simulink model "SimuPilot"  (R2024b)
settings: Solver=VariableStepAuto  StartTime=0.0  StopTime=10.0  RelTol=1e-3
undefined symbols (not defined in the file or in its folder): aspd_min, gravity, H_INIT, K_D, K_H, K_T, K_V, mass, PTCH2SRV_D, PTCH2SRV_RLL, PTCH2SRV_RMAX_DN, PTCH2SRV_RMAX_UP, PTCH2SRV_TCONST, PTCH_K_I, PTCH_K_P, RLL2SRV_D, RLL2SRV_MAX, RLL2SRV_TCONST, RLL_K_I, RLL_K_P, V_INIT, YAW2SRV_DAMP, YAW2SRV_INT, YAW2SRV_RLL, YAW2SRV_SLIP
settings Model: Creator=sh2323  LastModifiedBy=sh2323

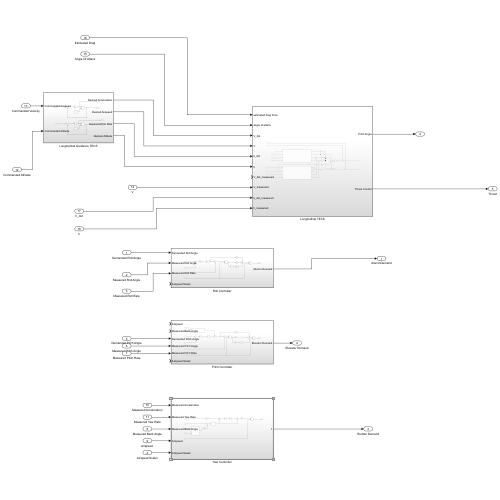
[thumbnail: Simulink's stored preview of the top-level diagram]
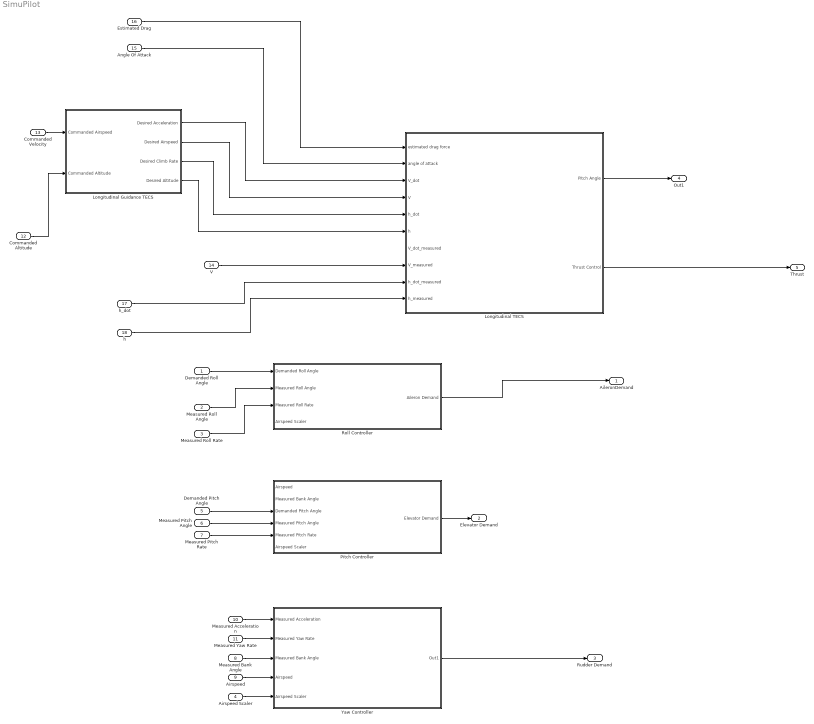
== system SimuPilot ==
  Demanded Roll Angle : Inport
  Measured Roll Angle : Inport  Port=2
  Measured Roll Rate : Inport  Port=3
  Airspeed Scaler : Inport  Port=4
  Demanded Pitch Angle : Inport  Port=5
  Measured Pitch Angle : Inport  Port=6
  Measured Pitch Rate : Inport  Port=7
  Measured Bank Angle : Inport  Port=8
  "Airspeed " : Inport  Port=9
  Measured Acceleration : Inport  Port=10
  Measured Yaw Rate : Inport  Port=11
  Commanded Altitude : Inport  Port=12
  Commanded Velocity : Inport  Port=13
  V : Inport  Port=14
  Angle Of Attack : Inport  Port=15
  Estimated Drag : Inport  Port=16
  h_dot : Inport  Port=17
  h : Inport  Port=18
  Longitudinal Guidance TECS : Subsystem
  Longitudinal TECS : Subsystem
  Pitch Controller : Subsystem
  Roll Controller : Subsystem
  Yaw Controller : Subsystem
  AileronDemand : Outport
  Elevator Demand : Outport  Port=2
  Rudder Demand : Outport  Port=3
  Out1 : Outport  Port=4
  Thrust : Outport  Port=5
  wires:
  Demanded Roll Angle/1 -> Roll Controller/1(Demanded Roll Angle)
  Measured Roll Angle/1 -> Roll Controller/2(Measured Roll Angle)
  Measured Roll Rate/1 -> Roll Controller/3(Measured Roll Rate)
  Roll Controller/1(Aileron Demand) -> AileronDemand/1
  Demanded Pitch Angle/1 -> Pitch Controller/3(Demanded Pitch Angle)
  Measured Pitch Angle/1 -> Pitch Controller/4(Measured Pitch Angle)
  Measured Pitch Rate/1 -> Pitch Controller/5(Measured Pitch Rate)
  Pitch Controller/1(Elevator Demand) -> Elevator Demand/1
  Measured Acceleration/1 -> Yaw Controller/1(Measured Acceleration)
  Measured Yaw Rate/1 -> Yaw Controller/2(Measured Yaw Rate)
  Measured Bank Angle/1 -> Yaw Controller/3(Measured Bank Angle)
  "Airspeed "/1 -> Yaw Controller/4(Airspeed)
  Airspeed Scaler/1 -> Yaw Controller/5(Airspeed Scaler)
  Yaw Controller/1(Out1) -> Rudder Demand/1
  Commanded Velocity/1 -> Longitudinal Guidance TECS/1(Commanded Airspeed)
  Commanded Altitude/1 -> Longitudinal Guidance TECS/2(Commanded Altitude)
  Estimated Drag/1 -> Longitudinal TECS/1(estimated drag force)
  Angle Of Attack/1 -> Longitudinal TECS/2(angle of attack)
  Longitudinal Guidance TECS/1(Desired Acceleration) -> Longitudinal TECS/3(V_dot)
  Longitudinal Guidance TECS/2(Desired Airspeed) -> Longitudinal TECS/4(V)
  Longitudinal Guidance TECS/3(Desired Climb Rate) -> Longitudinal TECS/5(h_dot)
  Longitudinal Guidance TECS/4(Desired Altitude) -> Longitudinal TECS/6(h)
  V/1 -> Longitudinal TECS/8(V_measured)
  h_dot/1 -> Longitudinal TECS/9(h_dot_measured)
  h/1 -> Longitudinal TECS/10(h_measured)
  Longitudinal TECS/1(Pitch Angle) -> Out1/1
  Longitudinal TECS/2(Thrust Control) -> Thrust/1

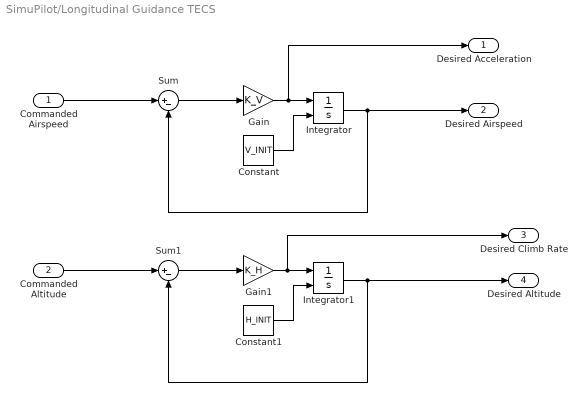
== system SimuPilot/Longitudinal Guidance TECS ==
  Commanded Airspeed : Inport
  Commanded Altitude : Inport  Port=2
  Constant : Constant  Value=V_INIT
  Constant1 : Constant  Value=H_INIT
  Gain : Gain  Gain=K_V
  Gain1 : Gain  Gain=K_H
  Integrator : Integrator  InitialConditionSource=external
  Integrator1 : Integrator  InitialConditionSource=external
  Sum : Sum  Inputs=|+-
  Sum1 : Sum  Inputs=|+-
  Desired Acceleration : Outport
  Desired Airspeed : Outport  Port=2
  Desired Climb Rate : Outport  Port=3
  Desired Altitude : Outport  Port=4
  wires:
  Sum/1 -> Gain/1
  Gain/1 -> Desired Acceleration/1, Integrator/1
  Commanded Altitude/1 -> Sum1/1
  Constant/1 -> Integrator/2
  Integrator1/1 -> Desired Altitude/1, Sum1/2
  Gain1/1 -> Desired Climb Rate/1, Integrator1/1
  Commanded Airspeed/1 -> Sum/1
  Integrator/1 -> Desired Airspeed/1, Sum/2
  Constant1/1 -> Integrator1/2
  Sum1/1 -> Gain1/1

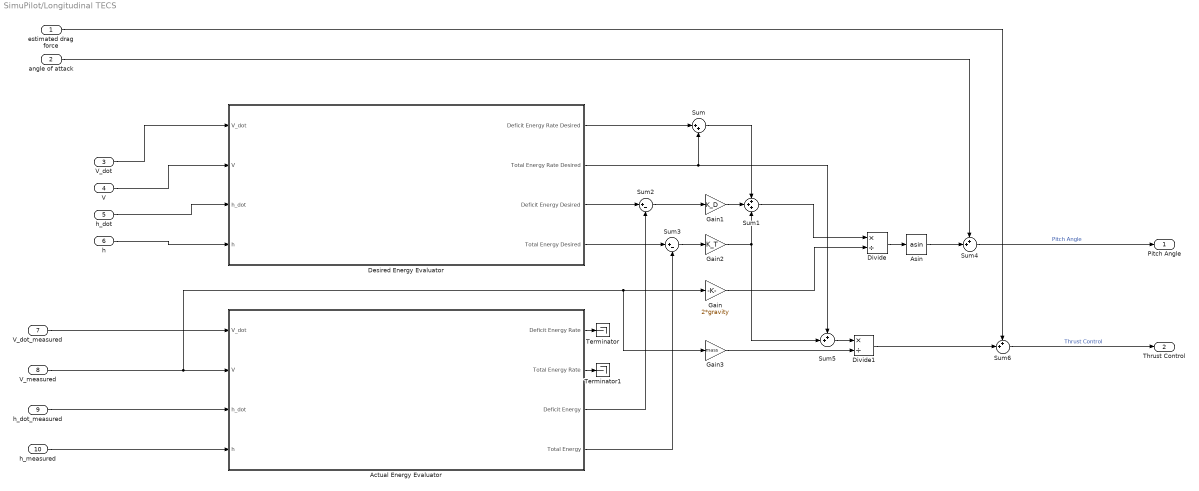
== system SimuPilot/Longitudinal TECS ==
  estimated drag force : Inport
  angle of attack : Inport  Port=2
  V_dot : Inport  Port=3
  V : Inport  Port=4
  h_dot : Inport  Port=5
  h : Inport  Port=6
  V_dot_measured : Inport  Port=7
  V_measured : Inport  Port=8
  h_dot_measured : Inport  Port=9
  h_measured : Inport  Port=10
  Actual Energy Evaluator : Subsystem
  Asin : Trigonometry  Operator=asin
  Desired Energy Evaluator : Subsystem
  Divide : Product  Inputs=*/
  Divide1 : Product  Inputs=*/
  Gain : Gain  Gain=2*gravity
  Gain1 : Gain  Gain=K_D
  Gain2 : Gain  Gain=K_T
  Gain3 : Gain  Gain=mass
  Sum : Sum  Inputs=|++
  Sum1 : Sum  Inputs=+++
  Sum2 : Sum  Inputs=|+-
  Sum3 : Sum  Inputs=|+-
  Sum4 : Sum  Inputs=++|
  Sum5 : Sum  Inputs=++|
  Sum6 : Sum  Inputs=++|
  Terminator : Terminator
  Terminator1 : Terminator
  Pitch Angle : Outport
  Thrust Control : Outport  Port=2
  wires:
  Desired Energy Evaluator/2(Total Energy Rate Desired) -> Sum5/1, Sum/2
  Divide/1 -> Asin/1
  Gain2/1 -> Sum5/2, Sum1/3
  angle of attack/1 -> Sum4/1
  Actual Energy Evaluator/3(Deficit Energy) -> Sum2/2
  V/1 -> Desired Energy Evaluator/2(V)
  Desired Energy Evaluator/3(Deficit Energy Desired) -> Sum2/1
  Sum3/1 -> Gain2/1
  V_measured/1 -> Gain3/1, Gain/1, Actual Energy Evaluator/2(V)
  Actual Energy Evaluator/4(Total Energy) -> Sum3/2
  h_dot_measured/1 -> Actual Energy Evaluator/3(h_dot)
  Sum/1 -> Sum1/1
  Gain/1 -> Divide/2
  Desired Energy Evaluator/1(Deficit Energy Rate Desired) -> Sum/1
  Gain3/1 -> Divide1/2
  Actual Energy Evaluator/1(Deficit Energy Rate) -> Terminator/1
  Divide1/1 -> Sum6/2
  Actual Energy Evaluator/2(Total Energy Rate) -> Terminator1/1
  h/1 -> Desired Energy Evaluator/4(h)
  Desired Energy Evaluator/4(Total Energy Desired) -> Sum3/1
  Sum5/1 -> Divide1/1
  Sum2/1 -> Gain1/1
  Asin/1 -> Sum4/2
  Gain1/1 -> Sum1/2
  Sum1/1 -> Divide/1
  V_dot_measured/1 -> Actual Energy Evaluator/1(V_dot)
  h_dot/1 -> Desired Energy Evaluator/3(h_dot)
  estimated drag force/1 -> Sum6/1
  V_dot/1 -> Desired Energy Evaluator/1(V_dot)
  Sum6/1 -> Thrust Control/1  "Thrust Control"
  h_measured/1 -> Actual Energy Evaluator/4(h)
  Sum4/1 -> Pitch Angle/1  "Pitch Angle"

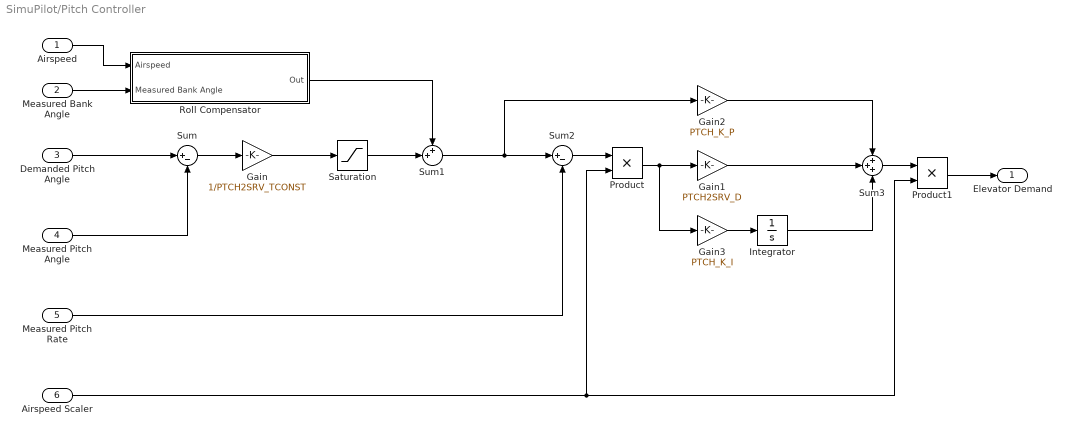
== system SimuPilot/Pitch Controller ==
  Airspeed : Inport
  Measured Bank Angle : Inport  Port=2
  Demanded Pitch Angle : Inport  Port=3
  Measured Pitch Angle : Inport  Port=4
  Measured Pitch Rate : Inport  Port=5
  Airspeed Scaler : Inport  Port=6
  Gain : Gain  Gain=1/PTCH2SRV_TCONST
  Gain1 : Gain  Gain=PTCH2SRV_D
  Gain2 : Gain  Gain=PTCH_K_P
  Gain3 : Gain  Gain=PTCH_K_I
  Integrator : Integrator
  Product : Product
  Product1 : Product
  Roll Compensator : Subsystem
  Saturation : Saturate  UpperLimit=PTCH2SRV_RMAX_UP  LowerLimit=PTCH2SRV_RMAX_DN
  Sum : Sum  Inputs=|+-
  Sum1 : Sum  Inputs=++|
  Sum2 : Sum  Inputs=|+-
  Sum3 : Sum  Inputs=+++
  Elevator Demand : Outport
  wires:
  Airspeed/1 -> Roll Compensator/1(Airspeed)
  Gain3/1 -> Integrator/1
  Gain1/1 -> Sum3/2
  Product1/1 -> Elevator Demand/1
  Measured Bank Angle/1 -> Roll Compensator/2(Measured Bank Angle)
  Sum3/1 -> Product1/1
  Measured Pitch Angle/1 -> Sum/2
  Saturation/1 -> Sum1/2
  Sum1/1 -> Gain2/1, Sum2/1
  Product/1 -> Gain3/1, Gain1/1
  Integrator/1 -> Sum3/3
  Demanded Pitch Angle/1 -> Sum/1
  Airspeed Scaler/1 -> Product1/2, Product/2
  Gain/1 -> Saturation/1
  Sum/1 -> Gain/1
  Sum2/1 -> Product/1
  Gain2/1 -> Sum3/1
  Roll Compensator/1(Out) -> Sum1/1
  Measured Pitch Rate/1 -> Sum2/2

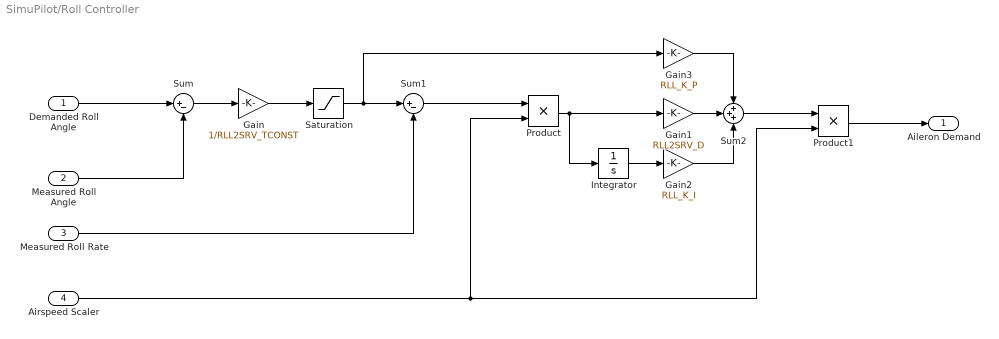
== system SimuPilot/Roll Controller ==
  Demanded Roll Angle : Inport
  Measured Roll Angle : Inport  Port=2
  Measured Roll Rate : Inport  Port=3
  Airspeed Scaler : Inport  Port=4
  Gain : Gain  Gain=1/RLL2SRV_TCONST
  Gain1 : Gain  Gain=RLL2SRV_D
  Gain2 : Gain  Gain=RLL_K_I
  Gain3 : Gain  Gain=RLL_K_P
  Integrator : Integrator
  Product : Product
  Product1 : Product
  Saturation : Saturate  UpperLimit=RLL2SRV_MAX  LowerLimit=-RLL2SRV_MAX
  Sum : Sum  Inputs=|+-
  Sum1 : Sum  Inputs=|+-
  Sum2 : Sum  Inputs=+++
  Aileron Demand : Outport
  wires:
  Product/1 -> Integrator/1, Gain1/1
  Sum/1 -> Gain/1
  Saturation/1 -> Sum1/1, Gain3/1
  Gain1/1 -> Sum2/2
  Integrator/1 -> Gain2/1
  Sum2/1 -> Product1/1
  Sum1/1 -> Product/1
  Gain/1 -> Saturation/1
  Gain3/1 -> Sum2/1
  Airspeed Scaler/1 -> Product1/2, Product/2
  Gain2/1 -> Sum2/3
  Demanded Roll Angle/1 -> Sum/1
  Measured Roll Angle/1 -> Sum/2
  Product1/1 -> Aileron Demand/1
  Measured Roll Rate/1 -> Sum1/2

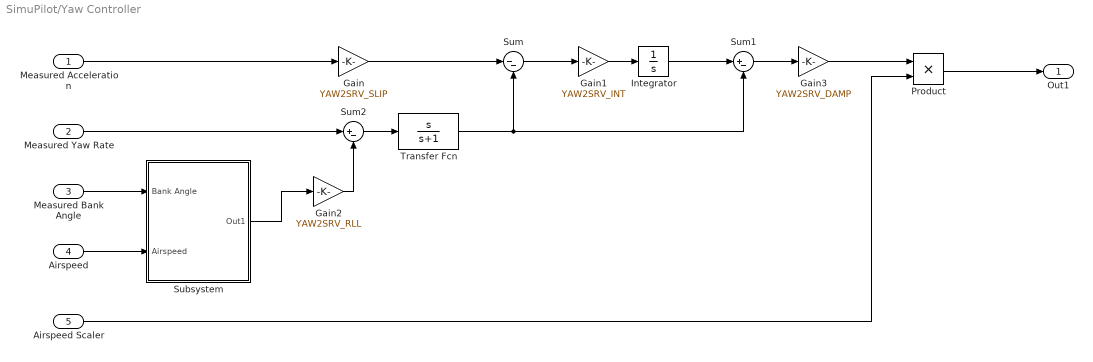
== system SimuPilot/Yaw Controller ==
  Measured Acceleration : Inport
  Measured Yaw Rate : Inport  Port=2
  Measured Bank Angle : Inport  Port=3
  Airspeed : Inport  Port=4
  Airspeed Scaler : Inport  Port=5
  Gain : Gain  Gain=YAW2SRV_SLIP
  Gain1 : Gain  Gain=YAW2SRV_INT
  Gain2 : Gain  Gain=YAW2SRV_RLL
  Gain3 : Gain  Gain=YAW2SRV_DAMP
  Integrator : Integrator
  Product : Product
  Subsystem : Subsystem
  Sum : Sum  Inputs=|--
  Sum1 : Sum  Inputs=|+-
  Sum2 : Sum  Inputs=|+-
  Transfer Fcn : TransferFcn  Numerator=[1 0]  Denominator=[1 1]
  Out1 : Outport
  wires:
  Sum1/1 -> Gain3/1
  Gain/1 -> Sum/1
  Gain3/1 -> Product/1
  Subsystem/1(Out1) -> Gain2/1
  Transfer Fcn/1 -> Sum1/2, Sum/2
  Sum/1 -> Gain1/1
  Integrator/1 -> Sum1/1
  Gain2/1 -> Sum2/2
  Measured Acceleration/1 -> Gain/1
  Sum2/1 -> Transfer Fcn/1
  Airspeed/1 -> Subsystem/2(Airspeed)
  Gain1/1 -> Integrator/1
  Measured Bank Angle/1 -> Subsystem/1(Bank Angle)
  Measured Yaw Rate/1 -> Sum2/1
  Airspeed Scaler/1 -> Product/2
  Product/1 -> Out1/1

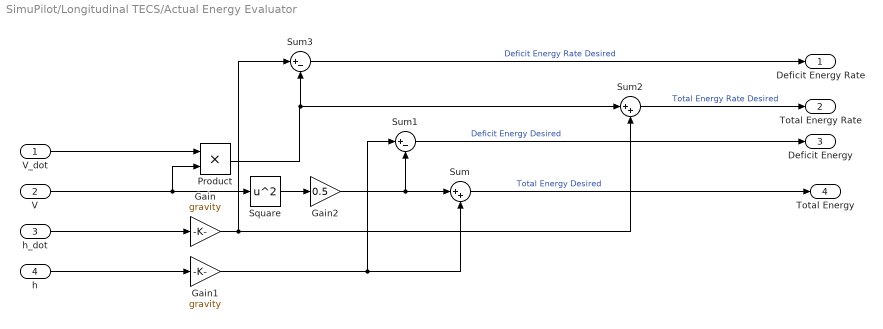
== system SimuPilot/Longitudinal TECS/Actual Energy Evaluator ==
  V_dot : Inport
  V : Inport  Port=2
  h_dot : Inport  Port=3
  h : Inport  Port=4
  Gain : Gain  Gain=gravity
  Gain1 : Gain  Gain=gravity
  Gain2 : Gain  Gain=0.5
  Product : Product
  Square : Math  Operator=square
  Sum : Sum  Inputs=|++
  Sum1 : Sum  Inputs=|+-
  Sum2 : Sum  Inputs=|++
  Sum3 : Sum  Inputs=|+-
  Deficit Energy Rate : Outport
  Total Energy Rate : Outport  Port=2
  Deficit Energy : Outport  Port=3
  Total Energy : Outport  Port=4
  wires:
  Gain2/1 -> Sum1/2, Sum/1
  Gain/1 -> Sum3/1, Sum2/2
  Square/1 -> Gain2/1
  Gain1/1 -> Sum1/1, Sum/2
  Product/1 -> Sum2/1, Sum3/2
  V/1 -> Product/2, Square/1
  Sum1/1 -> Deficit Energy/1  "Deficit Energy Desired"
  V_dot/1 -> Product/1
  h_dot/1 -> Gain/1
  h/1 -> Gain1/1
  Sum2/1 -> Total Energy Rate/1  "Total Energy Rate Desired"
  Sum/1 -> Total Energy/1  "Total Energy Desired"
  Sum3/1 -> Deficit Energy Rate/1  "Deficit Energy Rate Desired"

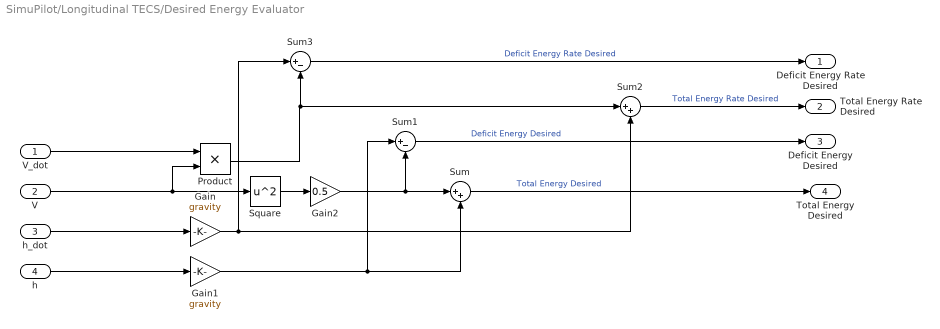
== system SimuPilot/Longitudinal TECS/Desired Energy Evaluator ==
  V_dot : Inport
  V : Inport  Port=2
  h_dot : Inport  Port=3
  h : Inport  Port=4
  Gain : Gain  Gain=gravity
  Gain1 : Gain  Gain=gravity
  Gain2 : Gain  Gain=0.5
  Product : Product
  Square : Math  Operator=square
  Sum : Sum  Inputs=|++
  Sum1 : Sum  Inputs=|+-
  Sum2 : Sum  Inputs=|++
  Sum3 : Sum  Inputs=|+-
  Deficit Energy Rate Desired : Outport
  Total Energy Rate Desired : Outport  Port=2
  Deficit Energy Desired : Outport  Port=3
  Total Energy Desired : Outport  Port=4
  wires:
  Gain2/1 -> Sum1/2, Sum/1
  Gain/1 -> Sum3/1, Sum2/2
  Square/1 -> Gain2/1
  Gain1/1 -> Sum1/1, Sum/2
  Product/1 -> Sum2/1, Sum3/2
  V/1 -> Product/2, Square/1
  Sum1/1 -> Deficit Energy Desired/1  "Deficit Energy Desired"
  V_dot/1 -> Product/1
  h_dot/1 -> Gain/1
  h/1 -> Gain1/1
  Sum2/1 -> Total Energy Rate Desired/1  "Total Energy Rate Desired"
  Sum/1 -> Total Energy Desired/1  "Total Energy Desired"
  Sum3/1 -> Deficit Energy Rate Desired/1  "Deficit Energy Rate Desired"

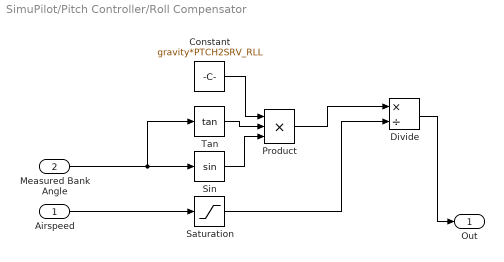
== system SimuPilot/Pitch Controller/Roll Compensator ==
  Airspeed : Inport
  Measured Bank Angle : Inport  Port=2
  Constant : Constant  Value=gravity*PTCH2SRV_RLL
  Divide : Product  Inputs=*/
  Product : Product  Inputs=3
  Saturation : Saturate  UpperLimit=inf  LowerLimit=aspd_min
  Sin : Trigonometry
  Tan : Trigonometry  Operator=tan
  Out : Outport
  wires:
  Measured Bank Angle/1 -> Tan/1, Sin/1
  Divide/1 -> Out/1
  Product/1 -> Divide/1
  Tan/1 -> Product/2
  Sin/1 -> Product/3
  Constant/1 -> Product/1
  Airspeed/1 -> Saturation/1
  Saturation/1 -> Divide/2

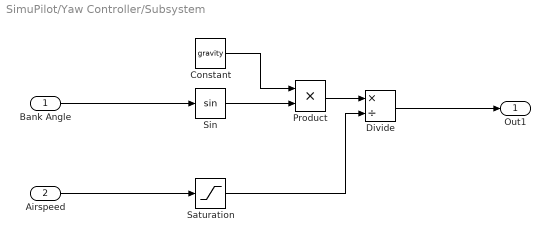
== system SimuPilot/Yaw Controller/Subsystem ==
  Bank Angle : Inport
  Airspeed : Inport  Port=2
  Constant : Constant  Value=gravity
  Divide : Product  Inputs=*/
  Product : Product
  Saturation : Saturate  UpperLimit=inf  LowerLimit=aspd_min
  Sin : Trigonometry
  Out1 : Outport
  wires:
  Divide/1 -> Out1/1
  Bank Angle/1 -> Sin/1
  Sin/1 -> Product/2
  Constant/1 -> Product/1
  Product/1 -> Divide/1
  Airspeed/1 -> Saturation/1
  Saturation/1 -> Divide/2
